simulink model "Encryption"  (R2024b)
settings: Solver=FixedStepAuto  StartTime=0.0  StopTime=10.0  RelTol=1e-3
libraries: androidcommunicationlib x2, androidaudiovideolib x1, dspsrcs4 x1
settings Model: Creator=Tarun  LastModifiedBy=tamiz
settings OptimizationCC: EnhancedBackFolding=on  PassReuseOutputArgsThreshold=0  MaxStackSize=64  OptimizeBlockOrder=speed  DifferentSizesBufferReuse=on  OptimizationCustomize=off
settings DebuggingCC: ParameterTunabilityLossMsg=error
settings HardwareCC: ProdBitPerLong=64  ProdLargestAtomicInteger=LongLong  ProdLargestAtomicFloat=Double  ProdLongLongMode=on  ProdHWDeviceType=ARM Compatible->ARM Cortex-A (64-bit)  UseEmbeddedCoderFeatures=off  UseSimulinkCoderFeatures=off
settings SFSimCC: MATLABDynamicMemAlloc=off
settings RTWCC: Description=Embedded Coder  SystemTargetFile=ert.tlc  HardwareBoard=Android Device (64bit)  TLCOptions="-aInlineSetEventsForThisBaseRateFcn=TLC_FALSE -aSuppressMultiTaskScheduler=TLC_FALSE  -aRateBasedStepFcn=0"  TemplateMakefile=ert_default_tmf  RTWVerbose=off  Toolchain=Android SDK/NDK Tools  GPUComputeCapability=3.5
settings CodeAppCC: ForceParamTrailComments=on  OperatorAnnotations=on
settings ERTTargetCC: ERTCustomFileBanners=off  SupportContinuousTime=on  SupportNonInlinedSFcns=on  RemoveResetFunc=off  ModelStepFunctionPrototypeControlCompliant=off  InlinedParameterPlacement=Hierarchical  DynamicArrayContainerType=coder::array

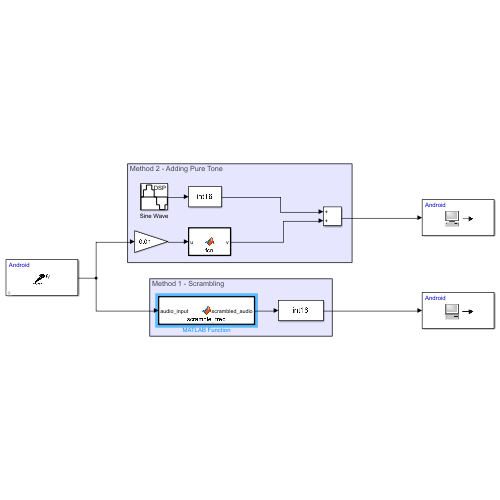
[thumbnail: Simulink's stored preview of the top-level diagram]
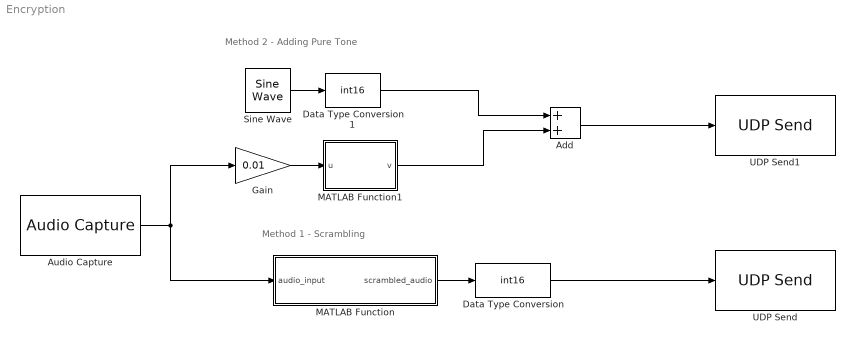
== system Encryption ==
  note: Method 2 - Adding Pure Tone
  note: Method 1 - Scrambling
  Add : Sum
  Audio Capture : androidaudiovideolib/Audio Capture  SampleFreq=44100  FrameSize=2205  SampleTime=0.05  SimulateUsing=Code generation  DeviceStr=0  QueueDuration=0  BlockPlatform=Android  AudioSamplingFreq=44100
  Data Type Conversion : DataTypeConversion  OutDataTypeStr=int16  SaturateOnIntegerOverflow=off  RndMeth=Floor
  Data Type Conversion1 : DataTypeConversion  OutDataTypeStr=int16  SaturateOnIntegerOverflow=off  RndMeth=Floor
  Gain : Gain  Gain=0.01
  MATLAB Function : MATLAB Function  TreatAsAtomicUnit=on
  MATLAB Function1 : MATLAB Function  TreatAsAtomicUnit=on
  Sine Wave : dspsrcs4/Sine Wave  Amplitude=5000  Frequency=10000  Phase=0  SampleMode=Discrete  OutComplex=Real  CompMethod=Trigonometric fcn  TableSize=Speed  SampleTime=1/44100  SamplesPerFrame=2205  ResetState=Restart at time zero  OutputFrames=off  dataType=double  wordLen=16  udDataType=sfix(16)  fracBitsMode=Best precision  numFracBits=15  OutDataTypeStr=double  LastOutDataTypeStr=double
  UDP Send : androidcommunicationlib/UDP Send  remoteURL='10.7.31.130'  remotePort=35000  localURL='0.0.0.0'  localPortSource=Automatically determine  localPort=-1  sampletime=-1  blockPlatform=Android  separateLengthPort=0
  UDP Send1 : androidcommunicationlib/UDP Send  remoteURL='10.7.31.130'  remotePort=36000  localURL='0.0.0.0'  localPortSource=Automatically determine  localPort=-1  sampletime=-1  blockPlatform=Android  separateLengthPort=0
  wires:
  Data Type Conversion/1 -> UDP Send/1
  MATLAB Function/1(scrambled_audio) -> Data Type Conversion/1
  Add/1 -> UDP Send1/1
  Audio Capture/1 -> MATLAB Function/1(audio_input), Gain/1
  Gain/1 -> MATLAB Function1/1(u)
  Sine Wave/1 -> Data Type Conversion1/1
  MATLAB Function1/1(v) -> Add/2
  Data Type Conversion1/1 -> Add/1

== matlab function Encryption/MATLAB Function ==
  data: audio_input input; scrambled_audio output
function scrambled_audio = scramble_freq(audio_input)
    seed=123;
    scrambled_audio = zeros(size(audio_input));
    rng(seed, 'twister');
    n = size(audio_input, 1);
    swap_indices = randperm(n);
    freq_audio_left = fft(audio_input(:,1));
    scrambled_freq_left = freq_audio_left(swap_indices);
    scrambled_audio(:,1) = real(ifft(scrambled_freq_left));
end

== matlab function Encryption/MATLAB Function1 ==
  data: u input; v output
function v = fcn(u)
    % u is an N x 2 matrix (stereo)
    % y will be an N x 1 matrix (mono, int16 type)

    % Average the two channels (left and right) to get a mono signal
    y = mean(u, 2);  % mean along the second dimension (columns)
    
    % Convert the result to int16 type
    v = int16(y);
end
